simulink library "ExampleComponent_v1"  (R2024b)
settings: Solver=FixedStepDiscrete  StartTime=0.0  StopTime=10.0  RelTol=1e-3
undefined symbols (not defined in the file or in its folder): Tsys
settings Model: Creator=Michael.Babst  LastModifiedBy=Michael.Babst
settings DebuggingCC: AlgebraicLoopMsg=error

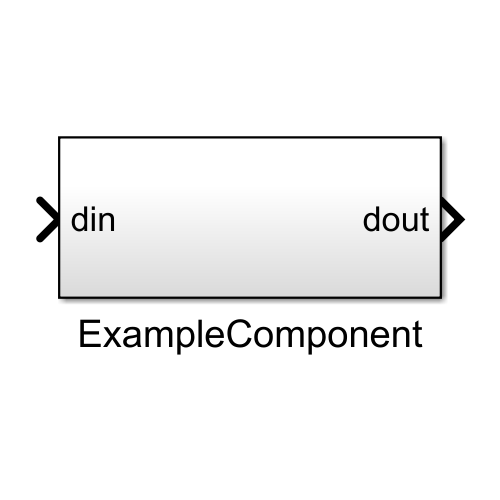
[thumbnail: Simulink's stored preview of the top-level diagram]
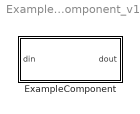
== system ExampleComponent_v1 ==
  ExampleComponent : Subsystem  mask{Tsys=Tsys}
      mask prompts: Tsys "System clock period"
      mask init:
      | ini = ExampleComponent_init(Tsys);
      settings: PermitHierarchicalResolution=None

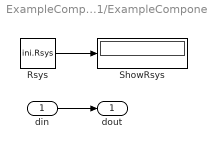
== system ExampleComponent_v1/ExampleComponent ==
  din : Inport
  Rsys : Constant  Value=ini.Rsys  SampleTime=Tsys
  ShowRsys : Display
  dout : Outport
  wires:
  Rsys/1 -> ShowRsys/1
  din/1 -> dout/1
